simulink model "sampleModel1604_sub_sub_sub"  (R2023a)
settings: Solver=VariableStepAuto  StartTime=0.0  StopTime=10.0  RelTol=1e-3
libraries: simulink x4, hdlsllib x3
settings Model: Creator=user1  LastModifiedBy=user1

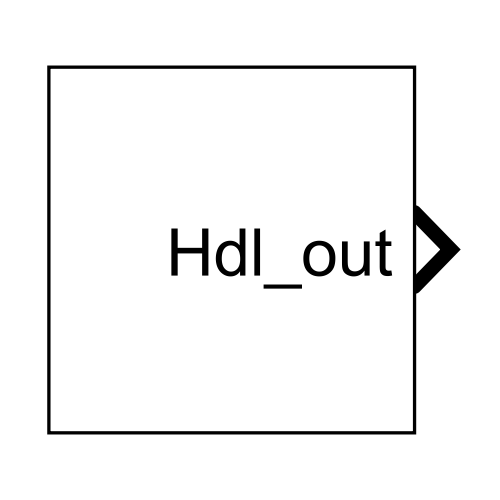
[thumbnail: Simulink's stored preview of the top-level diagram]
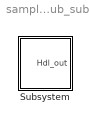
== system sampleModel1604_sub_sub_sub ==
  Subsystem : Subsystem

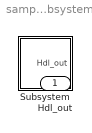
== system sampleModel1604_sub_sub_sub/Subsystem ==
  Subsystem : Subsystem
  Hdl_out : Outport  OutDataTypeStr=uint8

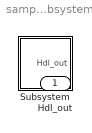
== system sampleModel1604_sub_sub_sub/Subsystem/Subsystem ==
  Subsystem : Subsystem
  Hdl_out : Outport  OutDataTypeStr=uint8

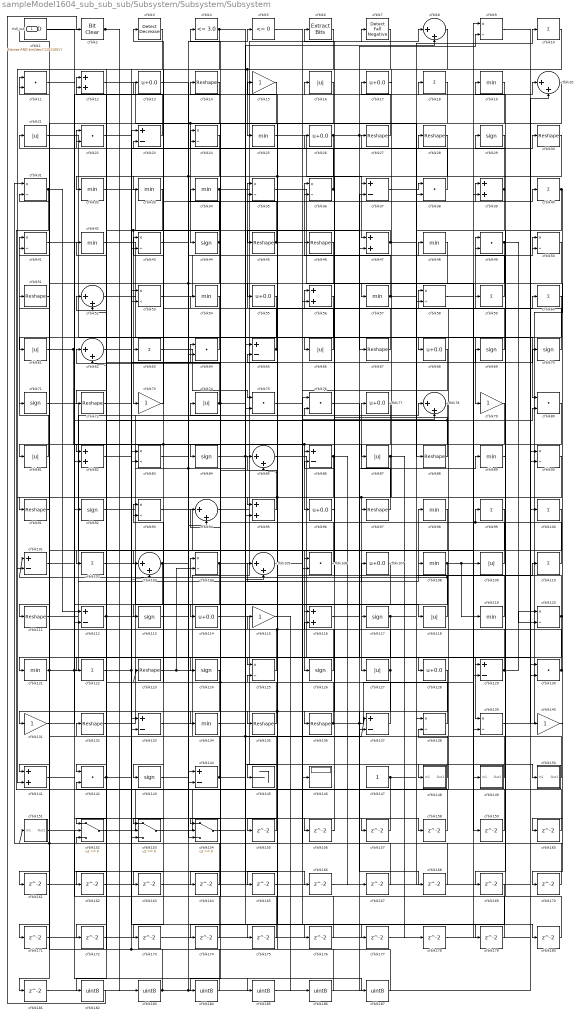
== system sampleModel1604_sub_sub_sub/Subsystem/Subsystem/Subsystem ==
  cfblk1 : simulink/Logic and Bit Operations/Bitwise Operator  logicop=AND  UseBitMask=on  BitMask=bin2dec('11011001')  BitMaskRealWorld=Stored Integer
      settings: LibrarySourceBlock=|
      | hdlsllib/Logic and Bit
      | Operations/Bitwise
      | Operator
  cfblk{10,18,40,59..60,63,99..100,102,110,122} (11 alike) : Sum  Inputs=+  OutDataTypeStr=uint8
  cfblk{23,37,65,86,101,112,129,133,137,144} (10 alike) : Sum  Inputs=+-  OutDataTypeStr=uint8
  cfblk{8,20,52,62,78,85,94,103,105} (9 alike) : Sum  Inputs=|++  OutDataTypeStr=uint8
  cfblk{9,24,31,35..36,41,43,50,53,58,83,90,93,104,120,125,138..139} (18 alike) : Product  Inputs=*/  OutDataTypeStr=uint8  RndMeth=Zero  SaturateOnIntegerOverflow=on
  cfblk{11,22,38,49,64,75..76,80,106,130,142} (11 alike) : DotProduct  OutDataTypeStr=uint8
  cfblk{13,17,26,55,68,77,96,107,114,128} (10 alike) : Bias  Bias=0.0  SaturateOnIntegerOverflow=off
  cfblk{19,25,32..34,42,48,54,57,89,98,108,119,121,134} (15 alike) : MinMax  OutDataTypeStr=uint8
  cfblk{16,21,61,66,74,81,87,109,118,127} (10 alike) : Abs  OutDataTypeStr=uint8  SaturateOnIntegerOverflow=off
  cfblk{14,27..28,30,45..46,51,67,72,88,91,97,111,123,132,135..136} (17 alike) : Reshape
  cfblk{29,44,69..71,84,92,113,117,124,126,143} (12 alike) : Signum
  cfblk{15,73,79,115,131,140} (6 alike) : Gain  OutDataTypeStr=uint8
  cfblk{12,39,47,56,82,95,116,141} (8 alike) : Sum  OutDataTypeStr=uint8
  cfblk145 : Terminator
  cfblk146 : Display
  cfblk147 : Constant  OutDataTypeStr=uint8  SampleTime=-1
  cfblk148 : Subsystem
      settings: LibrarySourceBlock=|
      | hdlsllib/Ports &
      | Subsystems/Subsystem
  cfblk149 : Subsystem
      settings: LibrarySourceBlock=|
      | hdlsllib/Ports &
      | Subsystems/Subsystem
  cfblk150 : Subsystem
      settings: LibrarySourceBlock=|
      | hdlsllib/Ports &
      | Subsystems/Subsystem
  cfblk151 : Subsystem
      settings: LibrarySourceBlock=|
      | hdlsllib/Ports &
      | Subsystems/Subsystem
  cfblk152 : Switch  OutDataTypeStr=uint8  SaturateOnIntegerOverflow=off  InputSameDT=off
  cfblk153 : Switch  OutDataTypeStr=uint8  SaturateOnIntegerOverflow=off  InputSameDT=off
  cfblk154 : Switch  OutDataTypeStr=uint8  SaturateOnIntegerOverflow=off  InputSameDT=off
  cfblk{155..181} (27 alike) : Delay  SampleTime=1
  cfblk{182..187} (6 alike) : DataTypeConversion  OutDataTypeStr=uint8  SaturateOnIntegerOverflow=off  RndMeth=Floor
  cfblk2 : simulink/Logic and Bit Operations/Bit Clear  iBit=0
      settings: LibrarySourceBlock=|
      | hdlsllib/Logic and Bit
      | Operations/Bit Clear
  cfblk3 : simulink/Logic and Bit Operations/Detect Decrease  vinit=0.0  OutDataTypeStr=uint8
      settings: LibrarySourceBlock=|
      | hdlsllib/Logic and Bit
      | Operations/Detect
      | Decrease
  cfblk4 : hdlsllib/Logic and Bit Operations/Compare To Constant  relop=<=  const=3.0  OutDataTypeStr=uint8
  cfblk5 : hdlsllib/Logic and Bit Operations/Compare To Zero  relop=<=  OutDataTypeStr=uint8
  cfblk6 : simulink/Logic and Bit Operations/Extract Bits  bitsToExtract=Upper half  numBits=8  bitIdxRange=[0 7]  outScalingMode=Preserve fixed-point scaling
      settings: LibrarySourceBlock=|
      | hdlsllib/Logic and Bit
      | Operations/Extract Bits
  cfblk7 : hdlsllib/Logic and Bit Operations/Detect Fall Negative  vinit=0  OutDataTypeStr=uint8
  Hdl_out : Outport  OutDataTypeStr=uint8
  wires:
  cfblk106/1 -> cfblk62/1
  cfblk114/1 -> cfblk148/1(In1)
  cfblk61/1 -> cfblk130/2, cfblk84/1
  cfblk96/1 -> cfblk104/1
  cfblk144/1 -> cfblk118/1, cfblk137/1, cfblk28/1
  cfblk94/1 -> cfblk16/1
  cfblk27/1 -> cfblk17/1
  cfblk81/1 -> cfblk41/1
  cfblk132/1 -> cfblk98/1
  cfblk93/1 -> cfblk126/1
  cfblk23/1 -> cfblk12/1
  cfblk149/1(Out1) -> cfblk108/1
  cfblk97/1 -> cfblk77/1
  cfblk104/1 -> cfblk172/1, cfblk60/1
  cfblk53/1 -> cfblk48/1
  cfblk33/1 -> cfblk53/2, cfblk73/1
  cfblk64/1 -> cfblk61/1
  cfblk139/1 -> cfblk57/1
  cfblk41/1 -> cfblk63/1
  cfblk123/1 -> cfblk104/2, cfblk78/1
  cfblk15/1 -> cfblk153/3, cfblk44/1
  cfblk21/1 -> cfblk79/1
  cfblk109/1 -> cfblk99/1, cfblk64/1
  cfblk88/1 -> cfblk22/2, cfblk6/1
  cfblk73/1 -> cfblk43/1
  cfblk87/1 -> cfblk178/1, cfblk113/1, cfblk127/1
  cfblk142/1 -> cfblk30/1, cfblk62/2
  cfblk136/1 -> cfblk93/2, cfblk168/1, cfblk9/1
  cfblk30/1 -> cfblk136/1
  cfblk119/1 -> cfblk56/1
  cfblk95/1 -> cfblk24/1
  cfblk137/1 -> cfblk42/1
  cfblk69/1 -> cfblk49/1
  cfblk86/1 -> cfblk167/1, cfblk165/1, cfblk101/2
  cfblk118/1 -> cfblk86/2, cfblk101/1
  cfblk133/1 -> cfblk39/1
  cfblk16/1 -> cfblk114/1
  cfblk125/1 -> cfblk52/1
  cfblk115/1 -> cfblk186/1
  cfblk113/1 -> cfblk50/1
  cfblk112/1 -> cfblk22/1, cfblk69/1
  cfblk12/1 -> cfblk88/1
  cfblk34/1 -> cfblk142/1, cfblk7/1
  cfblk108/1 -> cfblk163/1, cfblk119/1, cfblk109/1
  cfblk31/1 -> cfblk112/1, cfblk138/2
  cfblk8/1 -> cfblk97/1
  cfblk89/1 -> cfblk29/1
  cfblk19/1 -> cfblk134/1
  cfblk52/1 -> cfblk80/1
  cfblk76/1 -> cfblk128/1
  cfblk100/1 -> cfblk124/1
  cfblk13/1 -> cfblk144/1
  cfblk65/1 -> cfblk125/1, cfblk14/1
  cfblk84/1 -> cfblk50/2, cfblk8/1
  cfblk150/1(Out1) -> cfblk85/1
  cfblk121/1 -> cfblk11/2, cfblk80/2, cfblk76/2
  cfblk74/1 -> cfblk21/1, cfblk174/1, cfblk150/1(In1), cfblk34/1
  cfblk35/1 -> cfblk149/1(In1)
  cfblk138/1 -> cfblk74/1
  cfblk24/1 -> cfblk154/2, cfblk143/1
  cfblk83/1 -> cfblk20/1
  cfblk91/1 -> cfblk141/1
  cfblk85/1 -> cfblk139/1
  cfblk43/1 -> cfblk36/1
  cfblk28/1 -> cfblk47/1
  cfblk59/1 -> cfblk49/2
  cfblk57/1 -> cfblk40/1, cfblk36/2
  cfblk63/1 -> cfblk75/1
  cfblk26/1 -> cfblk56/2, cfblk9/2, cfblk68/1
  cfblk110/1 -> cfblk46/1
  cfblk42/1 -> cfblk140/1
  cfblk51/1 -> cfblk81/1
  cfblk117/1 -> cfblk59/1, cfblk122/1
  cfblk153/1 -> cfblk105/2
  cfblk17/1 -> cfblk87/1
  cfblk66/1 -> cfblk35/1
  cfblk140/1 -> cfblk31/1
  cfblk40/1 -> cfblk170/1, cfblk169/1
  cfblk78/1 -> cfblk153/1, cfblk91/1
  cfblk44/1 -> cfblk24/2, cfblk13/1, cfblk154/3, cfblk102/1
  cfblk50/1 -> cfblk55/1
  cfblk6/1 -> cfblk72/1, cfblk25/1
  cfblk102/1 -> cfblk117/1
  cfblk75/1 -> cfblk78/2
  cfblk46/1 -> cfblk95/1
  cfblk103/1 -> cfblk112/2, cfblk27/1
  cfblk143/1 -> cfblk5/1
  cfblk4/1 -> cfblk103/1, cfblk116/1
  cfblk20/1 -> cfblk121/1
  cfblk10/1 -> cfblk141/2
  cfblk37/1 -> cfblk38/1
  cfblk128/1 -> cfblk155/1, cfblk152/1
  cfblk45/1 -> cfblk177/1, cfblk35/2
  cfblk127/1 -> cfblk137/2, cfblk41/2
  cfblk72/1 -> cfblk70/1
  cfblk79/1 -> cfblk173/1, cfblk96/1
  cfblk147/1 -> cfblk142/2, cfblk110/1
  cfblk49/1 -> cfblk120/2, cfblk106/1
  cfblk98/1 -> cfblk145/1
  cfblk71/1 -> cfblk139/2
  cfblk55/1 -> cfblk95/2
  cfblk131/1 -> cfblk18/1
  cfblk3/1 -> cfblk83/2
  cfblk29/1 -> cfblk85/2, cfblk133/2
  cfblk36/1 -> cfblk11/1, cfblk66/1
  cfblk2/1 -> Hdl_out/1, cfblk183/1
  cfblk148/1(Out1) -> cfblk51/1
  cfblk62/1 -> cfblk86/1
  cfblk32/1 -> cfblk67/1
  cfblk135/1 -> cfblk123/1, cfblk4/1
  cfblk39/1 -> cfblk58/2, cfblk32/1
  cfblk120/1 -> cfblk54/1, cfblk131/1
  cfblk48/1 -> cfblk111/1
  cfblk122/1 -> cfblk179/1, cfblk103/2
  cfblk47/1 -> cfblk45/1, cfblk10/1
  cfblk9/1 -> cfblk130/1
  cfblk77/1 -> cfblk154/1
  cfblk111/1 -> cfblk107/1
  cfblk68/1 -> cfblk106/2
  cfblk152/1 -> cfblk94/2
  cfblk11/1 -> cfblk92/1
  cfblk7/1 -> cfblk33/1
  cfblk116/1 -> cfblk89/1
  cfblk5/1 -> cfblk146/1
  cfblk92/1 -> cfblk8/2, cfblk64/2
  cfblk90/1 -> cfblk135/1
  cfblk25/1 -> cfblk37/1
  cfblk129/1 -> cfblk120/1, cfblk93/1, cfblk65/2
  cfblk105/1 -> cfblk129/1
  cfblk67/1 -> cfblk23/2
  cfblk130/1 -> cfblk160/1, cfblk58/1
  cfblk54/1 -> cfblk82/1
  cfblk38/1 -> cfblk3/1
  cfblk14/1 -> cfblk82/2
  cfblk126/1 -> cfblk71/1
  cfblk70/1 -> cfblk26/1
  cfblk155/1 -> cfblk83/1
  cfblk141/1 -> cfblk156/1
  cfblk156/1 -> cfblk116/2
  cfblk82/1 -> cfblk157/1
  cfblk157/1 -> cfblk105/1
  cfblk154/1 -> cfblk158/1
  cfblk158/1 -> cfblk65/1
  cfblk58/1 -> cfblk159/1
  cfblk159/1 -> cfblk23/1
  cfblk160/1 -> cfblk125/2
  cfblk99/1 -> cfblk161/1
  cfblk161/1 -> cfblk75/2
  cfblk56/1 -> cfblk162/1
  cfblk162/1 -> cfblk43/2
  cfblk163/1 -> cfblk38/2
  cfblk107/1 -> cfblk164/1
  cfblk164/1 -> cfblk12/2
  cfblk165/1 -> cfblk138/1
  cfblk101/1 -> cfblk166/1
  cfblk166/1 -> cfblk20/2
  cfblk167/1 -> cfblk152/3
  cfblk168/1 -> cfblk76/1
  cfblk170/1 -> cfblk153/2
  cfblk60/1 -> cfblk171/1
  cfblk171/1 -> cfblk133/1
  cfblk172/1 -> cfblk129/2
  cfblk173/1 -> cfblk37/2
  cfblk174/1 -> cfblk152/2
  cfblk18/1 -> cfblk175/1
  cfblk175/1 -> cfblk94/1
  cfblk22/1 -> cfblk176/1
  cfblk176/1 -> cfblk52/2
  cfblk177/1 -> cfblk39/2
  cfblk178/1 -> cfblk90/2
  cfblk179/1 -> cfblk15/1
  cfblk134/1 -> cfblk180/1
  cfblk180/1 -> cfblk19/1
  cfblk124/1 -> cfblk181/1
  cfblk181/1 -> cfblk100/1
  cfblk80/1 -> cfblk182/1
  cfblk182/1 -> cfblk2/1
  cfblk183/1 -> cfblk31/2, cfblk151/1(In1), cfblk47/2, cfblk144/2
  cfblk169/1 -> cfblk184/1
  cfblk184/1 -> cfblk1/1
  cfblk1/1 -> cfblk185/1
  cfblk185/1 -> cfblk90/1
  cfblk186/1 -> cfblk132/1, cfblk53/1
  cfblk151/1(Out1) -> cfblk187/1
  cfblk187/1 -> cfblk115/1

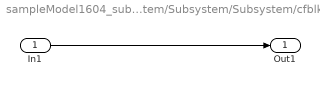
== system sampleModel1604_sub_sub_sub/Subsystem/Subsystem/Subsystem/cfblk148 ==
  In1 : Inport
  Out1 : Outport
  wires:
  In1/1 -> Out1/1

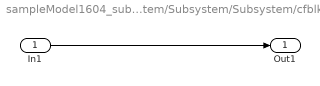
== system sampleModel1604_sub_sub_sub/Subsystem/Subsystem/Subsystem/cfblk149 ==
  In1 : Inport
  Out1 : Outport
  wires:
  In1/1 -> Out1/1

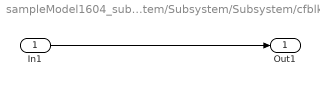
== system sampleModel1604_sub_sub_sub/Subsystem/Subsystem/Subsystem/cfblk150 ==
  In1 : Inport
  Out1 : Outport
  wires:
  In1/1 -> Out1/1

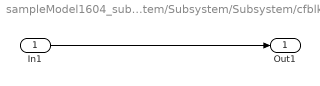
== system sampleModel1604_sub_sub_sub/Subsystem/Subsystem/Subsystem/cfblk151 ==
  In1 : Inport
  Out1 : Outport
  wires:
  In1/1 -> Out1/1
